simulink model "kfHdgSpdCtrl_2015b"  (R2015b)
settings: Solver=FixedStepAuto  StartTime=0.0  StopTime=inf  FixedStep=0.1  MaxStep=.1  RelTol=1e-3
undefined symbols (not defined in the file or in its folder): Left, Right
libraries: simulink_extras x7, robotlib x4, simulink x2, realtime_pacer_lib x1
settings Model: Creator=spkragel  LastModifiedBy=aschnieders22
settings ConfigComp: CovModelRefEnable=Off

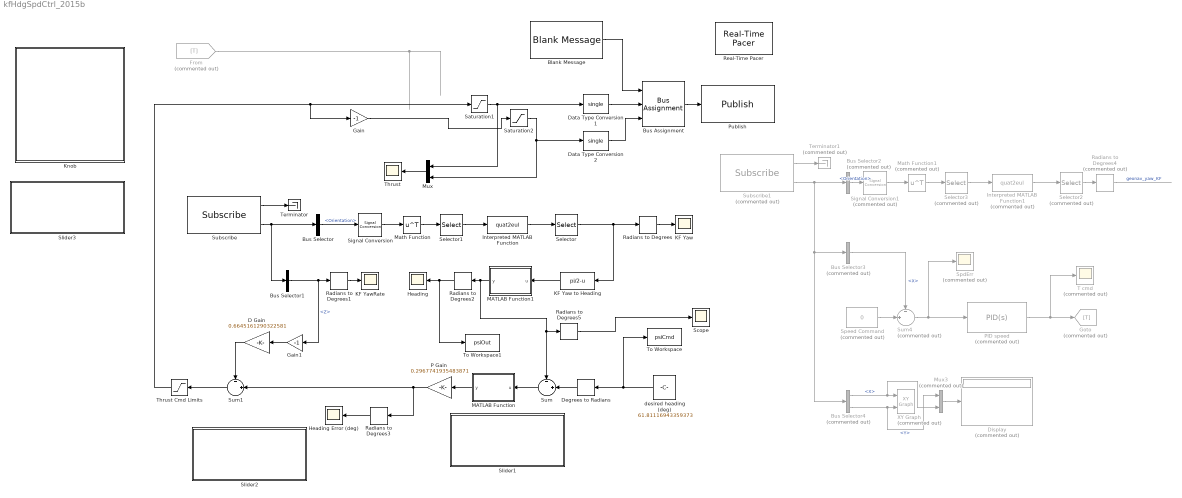
== system kfHdgSpdCtrl_2015b ==
  Blank Message : robotlib/Blank Message  SourceLibraryInfo=This block requires Robotics System Toolbox  messageType=kingfisher_msgs/Drive  SampleTime=inf
  Bus Assignment : BusAssignment  AssignedSignals=Left,Right
  Bus Selector : BusSelector  OutputSignals=Orientation
  Bus Selector1 : BusSelector  OutputSignals=AngularVelocity.Z
  Bus Selector2 : BusSelector  Commented=on  OutputSignals=Pose.Pose.Orientation
  Bus Selector3 : BusSelector  Commented=on  OutputSignals=Twist.Twist.Linear.X
  Bus Selector4 : BusSelector  Commented=on  OutputSignals=Pose.Pose.Position.X,Pose.Pose.Position.Y
  D Gain : Gain  Gain=0.6645161290322581
  Data Type Conversion1 : DataTypeConversion  OutDataTypeStr=single
  Data Type Conversion2 : DataTypeConversion  OutDataTypeStr=single
  Degrees to Radians : simulink_extras/Transformations/Degrees to Radians
  Display : Display  Commented=on
  From : From  Commented=on  GotoTag=T
  Gain : Gain  Gain=-1
  Gain1 : Gain  Gain=-1
  Goto : Goto  Commented=on  GotoTag=T
  Heading : Scope
  Heading Error (deg) : Scope
  Interpreted MATLAB Function : MATLABFcn  MATLABFcn=quat2eul  OutputDimensions=3
  Interpreted MATLAB Function1 : MATLABFcn  Commented=on  MATLABFcn=quat2eul  OutputDimensions=3
  KF Yaw : Scope
  KF Yaw to Heading : Fcn  Expr=pi/2-u
  KF YawRate : Scope
  Knob : Subsystem  DialogController=hmiCreateDDGDialog  IsWebBlock=on  mask(MWDashboardBlock){webBlockId=678e3d23-f724-4fd0-8e2d-7cce4adbba2a, webBlockType=continuousknob, ShowInLibBrowser=on, ShowInitialText=on, HMISrcModelName=kfHdgSpdCtrl_2015b}
      mask prompts: webBlockId "WebBlock Id"; webBlockType "WebBlock Type"; HMISrcModelName "Source Model"
      mask Help: helpview([docroot '/mapfiles/simulink.map'], 'hmi_knob')
      mask Display:
      | if strcmp(get_param(bdroot(gcb),'BlockDiagramType'), 'library')
      |     image([(matlabroot) '/toolbox/simulink/hmi/icons/ContinuousKnob.png']);
      | end
  MATLAB Function : MATLAB Function  TreatAsAtomicUnit=on
  MATLAB Function1 : MATLAB Function  TreatAsAtomicUnit=on
  Math Function : Math  Operator=transpose  SaturateOnIntegerOverflow=on
  Math Function1 : Math  Commented=on  Operator=transpose  SaturateOnIntegerOverflow=on
  Mux : Mux  Inputs=2
  Mux3 : Mux  Commented=on  Inputs=2
  P Gain : Gain  Gain=0.2967741935483871
  PID speed : simulink/Continuous/PID Controller  Commented=on  Controller=PID  TimeDomain=Continuous-time  SampleTime=-1  IntegratorMethod=Forward Euler  FilterMethod=Forward Euler  Form=Parallel  UseFilter=on  ControllerParametersSource=internal  P=1  I=2.5  D=0  N=100  InitialConditionSource=internal  InitialConditionForIntegrator=0  InitialConditionForFilter=0  ExternalReset=none  LimitOutput=on  UpperSaturationLimit=1  LowerSaturationLimit=-1  LinearizeAsGain=on  AntiWindupMode=clamping  Kb=1  TrackingMode=off  Kt=1  PParamMin=[]  PParamMax=[]  IParamMin=[]  IParamMax=[]  DParamMin=[]  DParamMax=[]  NParamMin=[]  NParamMax=[]  KbParamMin=[]  KbParamMax=[]  KtParamMin=[]  KtParamMax=[]  POutMin=[]  POutMax=[]  IOutMin=[]  IOutMax=[]  DOutMin=[]  DOutMax=[]  NOutMin=[]  NOutMax=[]  KbOutMin=[]  KbOutMax=[]  KtOutMin=[]  KtOutMax=[]  IntegratorOutMin=[]  IntegratorOutMax=[]  FilterOutMin=[]  FilterOutMax=[]  SumOutMin=[]  SumOutMax=[]  SumI1OutMin=[]  SumI1OutMax=[]  SumI2OutMin=[]  SumI2OutMax=[]  SumI3OutMin=[]  SumI3OutMax=[]  SumDOutMin=[]  SumDOutMax=[]  SaturationOutMin=[]  SaturationOutMax=[]  IntegratorContinuousStateAttributes=''  IntegratorStateMustResolveToSignalObject=off  IntegratorRTWStateStorageClass=Auto  FilterContinuousStateAttributes=''  FilterStateMustResolveToSignalObject=off  FilterRTWStateStorageClass=Auto  DifferentiatorICPrevScaledInput=0  DifferentiatorOutMin=[]  DifferentiatorOutMax=[]
  Publish : robotlib/Publish  SourceLibraryInfo=This block requires Robotics System Toolbox  topicSource=Select from ROS network  topic=/cmd_drive  messageType=kingfisher_msgs/Drive  messageQueueLength=1
  Radians to Degrees{,1..3,5} (5 alike) : simulink_extras/Transformations/Radians to Degrees
  Radians to Degrees4 : simulink_extras/Transformations/Radians to Degrees  Commented=on
  Real-Time Pacer : realtime_pacer_lib/Real-Time Pacer  simTimePerRealTime=1
  Saturation1 : Saturate  UpperLimit=1  LowerLimit=-1
  Saturation2 : Saturate  UpperLimit=1  LowerLimit=-1
  Scope : Scope
  Selector : Selector  InputPortWidth=3  IndexOptions=Index vector (dialog)  Indices=1  OutputSizes=1
  Selector1 : Selector  InputPortWidth=4  IndexOptions=Index vector (dialog)  Indices=[4 1 2 3]  OutputSizes=1
  Selector2 : Selector  Commented=on  InputPortWidth=3  IndexOptions=Index vector (dialog)  Indices=1  OutputSizes=1
  Selector3 : Selector  Commented=on  InputPortWidth=4  IndexOptions=Index vector (dialog)  Indices=[4 1 2 3]  OutputSizes=1
  Signal Conversion : SignalConversion  ConversionOutput=Virtual bus
  Signal Conversion1 : SignalConversion  Commented=on  ConversionOutput=Virtual bus
  Slider1 : Subsystem  DialogController=hmiCreateDDGDialog  IsWebBlock=on  mask(MWDashboardBlock){webBlockId=4eb0b11d-198b-4ea7-9d33-7fd3608c7df0, webBlockType=slider, ShowInLibBrowser=on, ShowInitialText=on, HMISrcModelName=kfHdgSpdCtrl_2015b}
      mask prompts: webBlockId "WebBlock Id"; webBlockType "WebBlock Type"; HMISrcModelName "Source Model"
      mask Help: helpview([docroot '/mapfiles/simulink.map'], 'hmi_slider')
      mask Display:
      | if strcmp(get_param(bdroot(gcb),'BlockDiagramType'), 'library')
      |     image([(matlabroot) '/toolbox/simulink/hmi/icons/Slider.png']);
      | end
  Slider2 : Subsystem  DialogController=hmiCreateDDGDialog  IsWebBlock=on  mask(MWDashboardBlock){webBlockId=d9dcd3fe-332f-4807-9693-eaf4deedbbd6, webBlockType=slider, ShowInLibBrowser=on, ShowInitialText=on, HMISrcModelName=kfHdgSpdCtrl_2015b}
      mask prompts: webBlockId "WebBlock Id"; webBlockType "WebBlock Type"; HMISrcModelName "Source Model"
      mask Help: helpview([docroot '/mapfiles/simulink.map'], 'hmi_slider')
      mask Display:
      | if strcmp(get_param(bdroot(gcb),'BlockDiagramType'), 'library')
      |     image([(matlabroot) '/toolbox/simulink/hmi/icons/Slider.png']);
      | end
  Slider3 : Subsystem  DialogController=hmiCreateDDGDialog  IsWebBlock=on  mask(MWDashboardBlock){webBlockId=1b9283b9-a227-43c8-bed9-ed4e2885c2b3, webBlockType=slider, ShowInLibBrowser=on, ShowInitialText=on, HMISrcModelName=kfHdgSpdCtrl_2015b}
      mask prompts: webBlockId "WebBlock Id"; webBlockType "WebBlock Type"; HMISrcModelName "Source Model"
      mask Help: helpview([docroot '/mapfiles/simulink.map'], 'hmi_slider')
      mask Display:
      | if strcmp(get_param(bdroot(gcb),'BlockDiagramType'), 'library')
      |     image([(matlabroot) '/toolbox/simulink/hmi/icons/Slider.png']);
      | end
  SpdErr : Scope  Commented=on
  Speed Command : Constant  Commented=on  Value=0
  Subscribe : robotlib/Subscribe  SourceLibraryInfo=This block requires Robotics System Toolbox  topicSource=Select from ROS network  topic=/imu/data  messageType=sensor_msgs/Imu  sampleTime=-1  messageQueueLength=1
  Subscribe1 : robotlib/Subscribe  Commented=on  SourceLibraryInfo=This block requires Robotics System Toolbox  topicSource=Select from ROS network  topic=/geonav_odom  messageType=nav_msgs/Odometry  sampleTime=-1  messageQueueLength=1
  Sum : Sum  Inputs=-|+||
  Sum1 : Sum  Inputs=-|+||
  Sum4 : Sum  Commented=on  Inputs=-|+||
  T cmd : Scope  Commented=on
  Terminator : Terminator
  Terminator1 : Terminator  Commented=on
  Thrust : Scope
  Thrust Cmd Limits : Saturate  UpperLimit=1  LowerLimit=-1
  To Workspace : ToWorkspace  VariableName=psiCmd  SaveFormat=Timeseries  SampleTime=-1
  To Workspace1 : ToWorkspace  VariableName=psiOut  SaveFormat=Timeseries  SampleTime=-1
  XY Graph : simulink/Sinks/XY Graph  Commented=on  xmin=130  xmax=200  ymin=50  ymax=270  st=-1
  desired heading (deg) : Constant  Value=61.81116943359373
  wires:
  Bus Assignment/1 -> Publish/1
  Blank Message/1 -> Bus Assignment/1
  Sum1/1 -> Thrust Cmd Limits/1
  Subscribe/2 -> Bus Selector/1, Bus Selector1/1
  Subscribe/1 -> Terminator/1
  Bus Selector/1 -> Signal Conversion/1  "<Orientation>"
  Interpreted MATLAB Function/1 -> Selector/1
  Signal Conversion/1 -> Math Function/1
  Math Function/1 -> Selector1/1
  Selector1/1 -> Interpreted MATLAB Function/1
  Selector/1 -> Radians to Degrees/1, KF Yaw to Heading/1
  Mux/1 -> Thrust/1
  KF Yaw to Heading/1 -> MATLAB Function1/1(u)
  Bus Selector1/1 -> Gain1/1, Radians to Degrees1/1  "<Z>"
  Radians to Degrees1/1 -> KF YawRate/1
  Radians to Degrees2/1 -> To Workspace1/1, Heading/1
  Sum/1 -> MATLAB Function/1(u)
  desired heading (deg)/1 -> To Workspace/1, Degrees to Radians/1
  Degrees to Radians/1 -> Sum/2
  P Gain/1 -> Sum1/2, Radians to Degrees3/1
  Radians to Degrees3/1 -> Heading Error (deg)/1
  MATLAB Function/1(y) -> P Gain/1
  MATLAB Function1/1(y) -> Radians to Degrees5/1, Sum/1, Radians to Degrees2/1
  D Gain/1 -> Sum1/1
  Gain1/1 -> D Gain/1
  From/1 -> ?
  Data Type Conversion1/1 -> Bus Assignment/2
  Data Type Conversion2/1 -> Bus Assignment/3
  Thrust Cmd Limits/1 -> Saturation1/1, Gain/1
  Subscribe1/1 -> Terminator1/1
  Subscribe1/2 -> Bus Selector4/1, Bus Selector3/1, Bus Selector2/1
  Interpreted MATLAB Function1/1 -> Selector2/1
  Signal Conversion1/1 -> Math Function1/1
  Math Function1/1 -> Selector3/1
  Selector3/1 -> Interpreted MATLAB Function1/1
  Bus Selector2/1 -> Signal Conversion1/1  "<Orientation>"
  Selector2/1 -> Radians to Degrees4/1
  Radians to Degrees4/1 -> ?  "geonav_yaw_KF"
  Radians to Degrees/1 -> KF Yaw/1
  Bus Selector3/1 -> Sum4/1  "<X>"
  Sum4/1 -> SpdErr/1, PID speed/1
  Speed Command/1 -> Sum4/2
  PID speed/1 -> T cmd/1, Goto/1
  Saturation1/1 -> Mux/1, Data Type Conversion1/1
  Saturation2/1 -> Mux/2, Data Type Conversion2/1
  Bus Selector4/1 -> Mux3/2, XY Graph/1  "<X>"
  Bus Selector4/2 -> Mux3/1, XY Graph/2  "<Y>"
  Mux3/1 -> Display/1
  Gain/1 -> Saturation2/1
  Radians to Degrees5/1 -> Scope/1

== system kfHdgSpdCtrl_2015b/Knob ==

== system kfHdgSpdCtrl_2015b/Slider1 ==

== system kfHdgSpdCtrl_2015b/Slider2 ==

== system kfHdgSpdCtrl_2015b/Slider3 ==

== matlab function kfHdgSpdCtrl_2015b/MATLAB Function1 ==
  data: u input; y output
function y = wrapToPi(u)
%#codegen

while u > pi
    u = u - 2*pi;
end;

while u < -pi
    u = u + 2*pi;
end;

y = u;

== matlab function kfHdgSpdCtrl_2015b/MATLAB Function ==
  data: u input; y output
function y = wrapToPi(u)
%#codegen

while u > pi
    u = u - 2*pi;
end;

while u < -pi
    u = u + 2*pi;
end;

y = u;
